simulink model "UpDownCounterMultiSate"  (R2025a)
settings: Solver=VariableStepAuto  StartTime=0.0  StopTime=Inf  RelTol=1e-3
settings Model: Creator=Soochan Kim  LastModifiedBy=Soochan Kim
settings OptimizationCC: BlockReduction=off  ConditionallyExecuteInputs=off  DefaultParameterBehavior=Inlined
settings DebuggingCC: AlgebraicLoopMsg=error
settings HardwareCC: ProdBitPerPointer=32.0  ProdBitPerSizeT=32.0  ProdBitPerPtrDiffT=32.0  ProdLargestAtomicFloat=None  ProdIntDivRoundTo=Undefined  ProdEndianess=Unspecified  ProdWordSize=32.0  ProdHWDeviceType=ASIC/FPGA->ASIC/FPGA  TargetBitPerPointer=64.0  TargetBitPerSizeT=64.0  TargetBitPerPtrDiffT=64.0  TargetLongLongMode=on  TargetIntDivRoundTo=Zero  TargetEndianess=LittleEndian  TargetWordSize=64.0  TargetHWDeviceType=Custom Processor->MATLAB Host Computer  ProdEqTarget=off

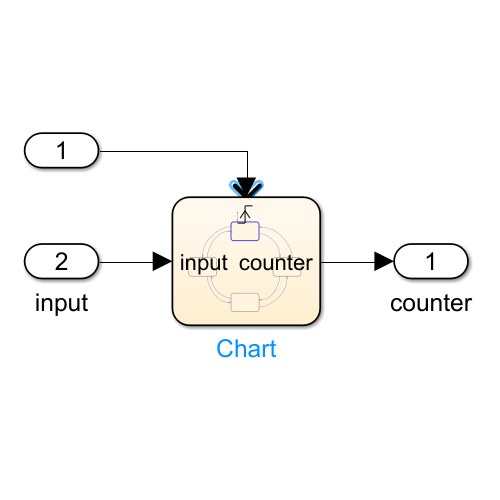
[thumbnail: Simulink's stored preview of the top-level diagram]
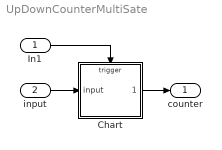
== system UpDownCounterMultiSate ==
  In1 : Inport  OutDataTypeStr=boolean
  input : Inport  Port=2  OutDataTypeStr=boolean
  Chart : Stateflow chart  TreatAsAtomicUnit=on
  counter : Outport  OutDataTypeStr=fixdt(0,2,0)  VectorParamsAs1DForOutWhenUnconnected=off
  wires:
  In1/1 -> Chart/Trigger
  input/1 -> Chart/1(input)
  Chart/1(counter) -> counter/1

== stateflow chart UpDownCounterMultiSate/Chart ==
  settings: executeAtInitialization=1
  state S01
    entry:
    counter=0;
  state S1
    entry:
    counter=1;
  state S3
    entry:
    counter=3;
  state S2
    entry:
    counter=2;
  (default) -> S01
  S3 -> S01 [order 1] : clk[input==1]
  S01 -> S1 [order 1] : clk[input==1]
  S1 -> S01 [order 2] : clk[input==0]
  S01 -> S3 [order 2] : clk[input==0]
  S1 -> S2 [order 1] : clk[input==1]
  S2 -> S1 [order 2] : clk [input==0]
  S2 -> S3 [order 1] : clk[input==1]
  S3 -> S2 [order 2] : clk [input==0]
  data: input input; counter output fixdt(0,2,0)
  events: clk input RISING_EDGE_EVENT
